simulink model "Autopilot"  (R2018b)
settings: Solver=ode45  StartTime=0.0  StopTime=5  RelTol=1e-3  AbsTol=1e-6
PreLoadFcn:
  | % aeroblk_init_HL20
  | aero_guid_dat
StopFcn:
  | aero_guid_plot
undefined symbols (not defined in the file): fin_max, fin_min
libraries: simulink_need_slupdate x6
settings Model: ExtModeTrigMode=oneshot  ExtModeArmWhenConnect=off  ExtModeAutoUpdateStatusClock=off  Creator=The MathWorks, Inc.  LastModifiedBy=smirsky
settings SolverCC: AutoScaleAbsTol=off  ZeroCrossAlgorithm=Adaptive  MinimalZcImpactIntegration=on
settings DataIOCC: SaveFormat=Array  SaveOutput=off  SaveTime=off  StateSaveName=xbase  OutputSaveName=ybase  SignalLoggingName=sigsOut
settings OptimizationCC: BlockReduction=off  ExpressionDepthLimit=2147483647  InitFltsAndDblsToZero=on  LifeSpan=inf
settings DebuggingCC: SaveWithParameterizedLinksMsg=none  SignalResolutionControl=None  MaxConsecutiveZCsMsg=none  MultiTaskDSMMsg=warning  MultiTaskCondExecSysMsg=none  SigSpecEnsureSampleTimeMsg=none  FcnCallInpInsideContextMsg=warning  StateNameClashWarn=warning  LibraryContextMissingDiagnostic=none  SFUnexpectedBacktrackingDiag=warning  SFNoUnconditionalDefaultTransitionDiag=warning  SFExecutionAtInitializationDiag=none
settings HardwareCC: ProdBitPerPointer=32  ProdBitPerSizeT=32  ProdBitPerPtrDiffT=32  ProdLargestAtomicFloat=None  ProdIntDivRoundTo=Undefined  ProdEndianess=Unspecified  ProdWordSize=32  ProdHWDeviceType=32-bit Generic
settings ModelReferenceCC: ModelReferenceNumInstancesAllowed=Single  PropagateSignalLabelsOutOfModel=off
settings SFSimCC: SimUseLocalCustomCode=off  SimParseCustomCode=off
settings RTWCC: RTWUseLocalCustomCode=off
settings CodeAppCC: StateflowObjectComments=on
settings GRTTargetCC: TargetFcnLib=ansi_tfl_tmw.mat  TargetLangStandard=C89/C90 (ANSI)  GeneratePreprocessorConditionals=Disable all  CombineOutputUpdateFcns=off  GRTInterface=on
settings ConfigComp: CovMetricSettings=d  CovHtmlReporting=on  CovSaveCumulativeToWorkspaceVar=on  CovSaveSingleToWorkspaceVar=on  CovExternalEMLEnable=off  CovSFcnEnable=off

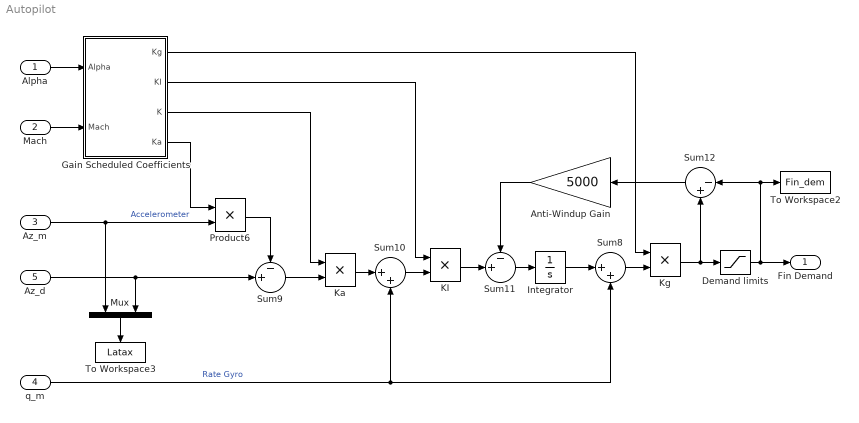
== system Autopilot ==
  Alpha : Inport  OutDataTypeStr=double  PortDimensions=1  SampleTime=0
  Mach : Inport  Port=2  OutDataTypeStr=double  PortDimensions=1  SampleTime=0
  Az_m : Inport  Port=3  OutDataTypeStr=double  PortDimensions=1  SampleTime=0
  q_m : Inport  Port=4  OutDataTypeStr=double  PortDimensions=1  SampleTime=0
  Az_d : Inport  Port=5  OutDataTypeStr=double  PortDimensions=1  SampleTime=0
  Anti-Windup Gain : Gain  Gain=5000  SaturateOnIntegerOverflow=on  OutDataTypeStr=Inherit: Same as input  ParamDataTypeStr=Inherit: Same as input
  "Demand limits " : Saturate  UpperLimit=fin_max  LowerLimit=fin_min
  Gain Scheduled Coefficients : Subsystem
  Integrator : Integrator
  KI : Product  SaturateOnIntegerOverflow=on  InputSameDT=on  OutDataTypeStr=Inherit: Same as first input
  Ka : Product  SaturateOnIntegerOverflow=on  InputSameDT=on  OutDataTypeStr=Inherit: Same as first input
  Kg : Product  SaturateOnIntegerOverflow=on  InputSameDT=on  OutDataTypeStr=Inherit: Same as first input
  Mux : Mux  Inputs=2
  Product6 : Product  SaturateOnIntegerOverflow=on  InputSameDT=on  OutDataTypeStr=Inherit: Same as first input
  Sum10 : Sum  Inputs=|++  SaturateOnIntegerOverflow=on  InputSameDT=on  OutDataTypeStr=Inherit: Same as first input
  Sum11 : Sum  Inputs=-+|  SaturateOnIntegerOverflow=on  InputSameDT=on  OutDataTypeStr=Inherit: Same as first input
  Sum12 : Sum  Inputs=|-+  SaturateOnIntegerOverflow=on  InputSameDT=on  OutDataTypeStr=Inherit: Same as first input
  Sum8 : Sum  Inputs=|++  SaturateOnIntegerOverflow=on  InputSameDT=on  OutDataTypeStr=Inherit: Same as first input
  Sum9 : Sum  Inputs=-+|  SaturateOnIntegerOverflow=on  InputSameDT=on  OutDataTypeStr=Inherit: Same as first input
  To Workspace2 : ToWorkspace  VariableName=Fin_dem  SaveFormat=Structure With Time  SampleTime=-1
  To Workspace3 : ToWorkspace  VariableName=Latax  SaveFormat=Structure With Time  SampleTime=-1
  Fin Demand : Outport  OutDataTypeStr=double  PortDimensions=1  SampleTime=0  InitialOutput=0
  wires:
  Mach/1 -> Gain Scheduled Coefficients/2(Mach)
  Alpha/1 -> Gain Scheduled Coefficients/1(Alpha)
  Kg/1 -> "Demand limits "/1, Sum12/2
  Gain Scheduled Coefficients/1("Kg ") -> Kg/1
  Gain Scheduled Coefficients/3("K ") -> Ka/1
  Gain Scheduled Coefficients/2("KI ") -> KI/1
  Anti-Windup Gain/1 -> Sum11/1
  Sum8/1 -> Kg/2
  Integrator/1 -> Sum8/1
  Sum11/1 -> Integrator/1
  Product6/1 -> Sum9/1
  Sum9/1 -> Ka/2
  Ka/1 -> Sum10/1
  Sum10/1 -> KI/2
  KI/1 -> Sum11/2
  Sum12/1 -> Anti-Windup Gain/1
  Az_d/1 -> Sum9/2, Mux/2
  Mux/1 -> To Workspace3/1
  q_m/1 -> Sum8/2, Sum10/2  "Rate Gyro"
  "Demand limits "/1 -> To Workspace2/1, Sum12/1, Fin Demand/1
  Az_m/1 -> Product6/2, Mux/1  "Accelerometer"
  Gain Scheduled Coefficients/4("Ka ") -> Product6/1

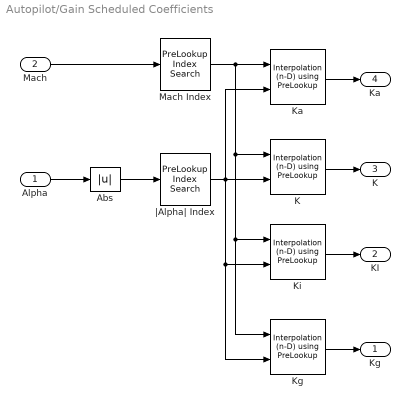
== system Autopilot/Gain Scheduled Coefficients ==
  Alpha : Inport
  Mach : Inport  Port=2
  Abs : Abs  SaturateOnIntegerOverflow=on
  K : simulink_need_slupdate/Interpolation (n-D) using PreLookup  numDimsPopupSelect=2  explicitNumDims=2  table=K  interpMethod=Linear  extrapMethod=Linear  rangeErrorMode=None  NumSelectionDims=0
      settings: SourceProductName=Simulink  SourceProductBaseCode=SL
  Ka : simulink_need_slupdate/Interpolation (n-D) using PreLookup  numDimsPopupSelect=2  explicitNumDims=2  table=Ka  interpMethod=Linear  extrapMethod=Linear  rangeErrorMode=None  NumSelectionDims=0
      settings: SourceProductName=Simulink  SourceProductBaseCode=SL
  Kg : simulink_need_slupdate/Interpolation (n-D) using PreLookup  numDimsPopupSelect=2  explicitNumDims=2  table=Kg  interpMethod=Linear  extrapMethod=Linear  rangeErrorMode=None  NumSelectionDims=0
      settings: SourceProductName=Simulink  SourceProductBaseCode=SL
  Ki : simulink_need_slupdate/Interpolation (n-D) using PreLookup  numDimsPopupSelect=2  explicitNumDims=2  table=Ki  interpMethod=Linear  extrapMethod=Linear  rangeErrorMode=None  NumSelectionDims=0
      settings: SourceProductName=Simulink  SourceProductBaseCode=SL
  Mach Index : simulink_need_slupdate/PreLookup Index Search  bpData=M_sch  searchMode=Binary Search  cacheBpFlag=on  outputFlag=off  IndexDataType=uint32  extrapMode=Linear Extrapolation  rangeErrorMode=None
      settings: SourceProductName=Simulink  SourceProductBaseCode=SL
  |Alpha| Index : simulink_need_slupdate/PreLookup Index Search  bpData=alpha_sch  searchMode=Binary Search  cacheBpFlag=on  outputFlag=off  IndexDataType=uint32  extrapMode=Linear Extrapolation  rangeErrorMode=None
      settings: SourceProductName=Simulink  SourceProductBaseCode=SL
  "Kg " : Outport  InitialOutput=0
  "KI " : Outport  Port=2  InitialOutput=0
  "K " : Outport  Port=3  InitialOutput=0
  "Ka " : Outport  Port=4  InitialOutput=0
  wires:
  Mach/1 -> Mach Index/1
  Abs/1 -> |Alpha| Index/1
  Kg/1 -> "Kg "/1
  Ki/1 -> "KI "/1
  K/1 -> "K "/1
  Ka/1 -> "Ka "/1
  |Alpha| Index/1 -> Ka/2, Kg/2, Ki/2, K/2
  Mach Index/1 -> Kg/1, Ki/1, K/1, Ka/1
  Alpha/1 -> Abs/1
